simulink library "JumpDetectionUint"  (R2020b)
settings: Solver=VariableStepAuto  StartTime=0.0  StopTime=10.0  RelTol=1e-3
settings Model: Creator=GW00166368  LastModifiedBy=GW00166368

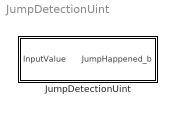
== system JumpDetectionUint ==
  JumpDetectionUint : Subsystem  mask(JumpDetectionUint){StartValue=0, FinishValue=0}
      mask help: 检测一个周期内，整形输入是否存在从StartValue到FinishValue的跳变，StartValue和FinishValue非整数时四舍五入取整。

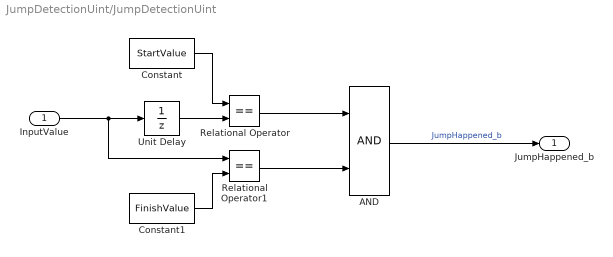
== system JumpDetectionUint/JumpDetectionUint ==
  InputValue : Inport  OutDataTypeStr=uint8
  AND : Logic  AllPortsSameDT=off  OutDataTypeStr=boolean
  Constant : Constant  Value=StartValue  OutDataTypeStr=uint8
  Constant1 : Constant  Value=FinishValue  OutDataTypeStr=uint8
  Relational Operator : RelationalOperator  Operator===  OutDataTypeStr=boolean  RndMeth=Simplest
  Relational Operator1 : RelationalOperator  Operator===  OutDataTypeStr=boolean  RndMeth=Simplest
  Unit Delay : UnitDelay  SampleTime=-1  HasFrameUpgradeWarning=on
  JumpHappened_b : Outport
  wires:
  Constant1/1 -> Relational Operator1/2
  Constant/1 -> Relational Operator/1
  AND/1 -> JumpHappened_b/1  "JumpHappened_b"
  Relational Operator1/1 -> AND/2
  Relational Operator/1 -> AND/1
  InputValue/1 -> Unit Delay/1, Relational Operator1/1
  Unit Delay/1 -> Relational Operator/2
